simulink model "hdlFrame_HistogramEqualization"  (R2023a)
settings: Solver=VariableStepAuto  StartTime=0.0  StopTime=3  RelTol=1e-3
undefined symbols (not defined in the file or in its folder): gray, Rec, SDTV
libraries: visionconversions x1, visionsources x1, visiongeotforms x1
settings Model: Creator=navan  LastModifiedBy=navan
settings SolverCC: MaxZcPerStep=1
settings OptimizationCC: BlockReduction=off  ConditionallyExecuteInputs=off  ReuseModelBlockBuffer=off
settings DebuggingCC: UnconnectedInputMsg=warning  UnconnectedOutputMsg=warning  UnconnectedLineMsg=warning  SFMachineParentedDataDiag=error
settings ModelReferenceCC: EnableRefExpFcnMdlSchedulingChecks=on
settings RTWCC: DLArmComputeVersion=19.05

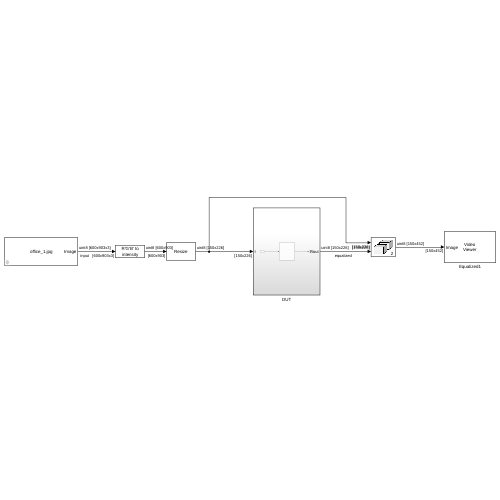
[thumbnail: Simulink's stored preview of the top-level diagram]
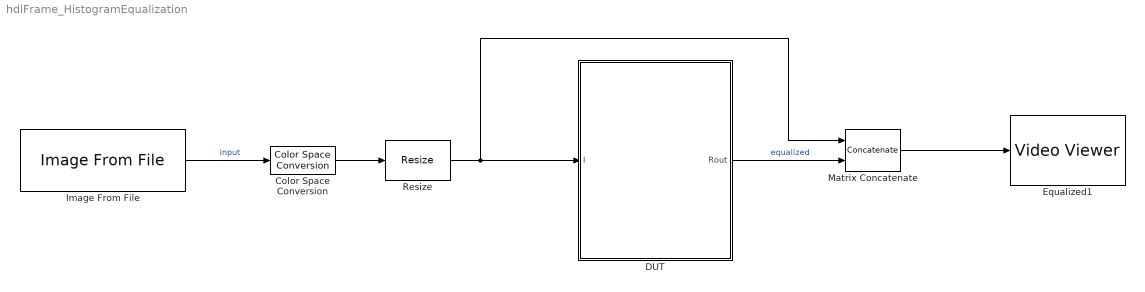
== system hdlFrame_HistogramEqualization ==
  Color Space Conversion : visionconversions/Color Space  Conversion  conversion=Obsolete  conversionActive=R'G'B' to intensity  wp_str=D65  rec=Rec. 601 (SDTV)  sys=1125/60/2:1  imagePorts=One multidimensional signal
  DUT : Subsystem
  Equalized1 : VideoViewer  colormapValue=gray(256)  FigPos=[151 944 936.666666666667 363]
  Image From File : visionsources/Image From File  Tag=vipblks_nd  FileName=office_1.jpg  Ts=1  imagePorts=One multidimensional signal  OutPortLabels=R|G|B  ImageDataType=uint8  sdImageDataType=uint(8)  Signed=on  WordLength=16  FractionLengthMode=User-defined  FractionLength=15
  Matrix Concatenate : Concatenate  Mode=Multidimensional array  ConcatenateDimension=2
  Resize : visiongeotforms/Resize  specify=Output size as a percentage of input size  rfactor=[25 25]  outCols=25  outRows=25  outRowsCols=[25 35]  interp_method=Bilinear  antialias=on  useROI=off  roiFlag=off  roundingMode=Nearest  overflowMode=on  prodOutputMode=Binary point scaling  prodOutputWordLength=32  prodOutputFracLength=10
  wires:
  Image From File/1 -> Color Space Conversion/1  "input"
  Matrix Concatenate/1 -> Equalized1/1
  DUT/1(Rout) -> Matrix Concatenate/2  "equalized"
  Resize/1 -> DUT/1(I), Matrix Concatenate/1
  Color Space Conversion/1 -> Resize/1

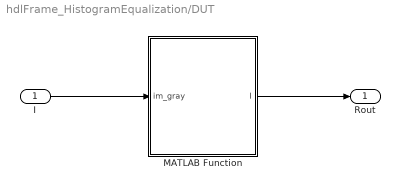
== system hdlFrame_HistogramEqualization/DUT ==
  I : Inport
  MATLAB Function : MATLAB Function  TreatAsAtomicUnit=on
  Rout : Outport
  wires:
  I/1 -> MATLAB Function/1(im_gray)
  MATLAB Function/1(I) -> Rout/1

== matlab function hdlFrame_HistogramEqualization/DUT/MATLAB Function ==
  data: im_gray input; I output
function I = histeq(im_gray)
% Uses single loop for post histogram processing to compute cdf

% histogram calculation
hist = zeros(1, 256, 'uint32');
hist = hdl.iteratorfun(@hist_kernel_fcn, im_gray, hist);

[row,col] = size(im_gray);
factor = coder.const(fi(255/(row*col)));

cdf_init = zeros(1,256,'uint8');
cdf = hdl.iteratorfun(@cdf_compute, hist, cdf_init, factor);

% Replacing the value from look up table
I = hdl.npufun(@table_lookup, [1,1], im_gray, 'NonSampleInput', cdf);

end

function count = hist_kernel_fcn(pix, count, idx) %#ok<INUSD> 

count(pix+1) = count(pix+1) +1;

end

function cdf = cdf_compute(hist, cdf, idx, factor)

if idx > 1
    cdf(idx) = uint8(cdf(idx-cast(1,'like',idx)) + hist*factor);
else
    cdf(1) = uint8(hist*factor);
end

end

function out = table_lookup(in, cdf)
    if in ~= 0
        out = cdf(in);
    else
        out = in;
    end
end
